simulink model "acquire_data_mag"  (R2017b)
settings: Solver=FixedStepDiscrete  StartTime=0.0  StopTime=10.0  RelTol=1e-3
undefined symbols (not defined in the file or in its folder): RGBLED_COLOR_ENUM, RGBLED_MODE_ENUM
libraries: pixhawk_slib_sensors_actuators x3
settings Model: Creator=Mr Wang  LastModifiedBy=Mr Wang
settings OptimizationCC: DefaultParameterBehavior=Inlined  MaxStackSize=128
settings DebuggingCC: ParameterTunabilityLossMsg=error
settings HardwareCC: ProdBitPerPointer=32  ProdBitPerSizeT=32  ProdBitPerPtrDiffT=32  ProdLargestAtomicInteger=Long  ProdLargestAtomicFloat=Double  ProdWordSize=32  ProdHWDeviceType=ARM Compatible->ARM Cortex
settings SFSimCC: MATLABDynamicMemAlloc=off
settings RTWCC: SystemTargetFile=ert.tlc  HardwareBoard=Pixhawk PX4  TemplateMakefile=ert_default_tmf  GenerateReport=on  Toolchain=Pixhawk Toolchain  IncludeHyperlinkInReport=on  LaunchReport=on  GenerateTraceInfo=on  GenerateTraceReport=on  GenerateTraceReportSl=on  GenerateTraceReportSf=on  GenerateTraceReportEml=on
settings CodeAppCC: ForceParamTrailComments=on  IgnoreCustomStorageClasses=off  OperatorAnnotations=on  SimulinkDataObjDesc=on  SFDataObjDesc=on  MATLABFcnDesc=on  InsertBlockDesc=on  StateflowObjectComments=on  MATLABSourceComments=on
settings ERTTargetCC: MultiwordLength=2048  ERTCustomFileTemplate=PX4_codertarget_file_process.tlc

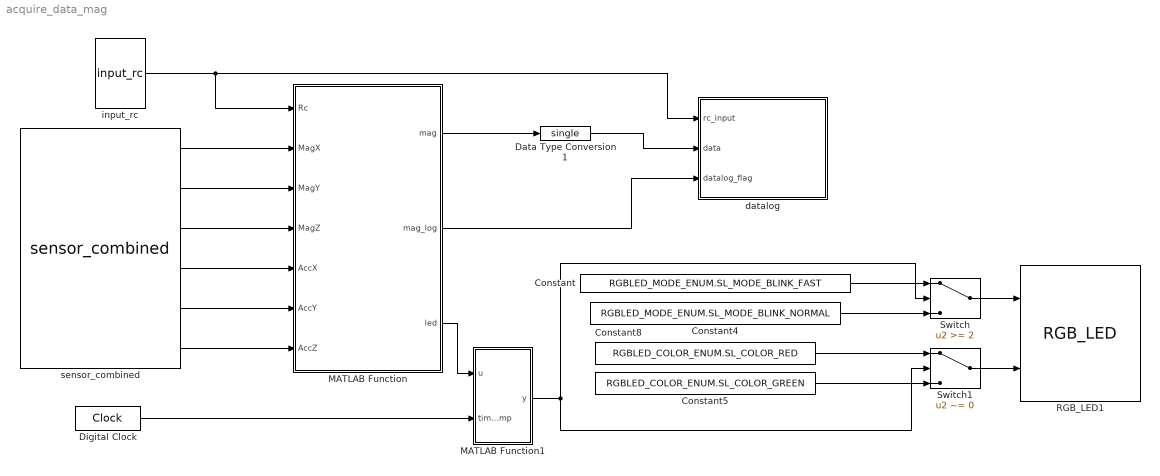
== system acquire_data_mag ==
  Constant : Constant  Value=RGBLED_MODE_ENUM.SL_MODE_BLINK_FAST  OutDataTypeStr=Enum: RGBLED_MODE_ENUM
  Constant4 : Constant  Value=RGBLED_MODE_ENUM.SL_MODE_BLINK_NORMAL  OutDataTypeStr=Enum: RGBLED_MODE_ENUM
  Constant5 : Constant  Value=RGBLED_COLOR_ENUM.SL_COLOR_GREEN  OutDataTypeStr=Enum: RGBLED_COLOR_ENUM
  Constant8 : Constant  Value=RGBLED_COLOR_ENUM.SL_COLOR_RED  OutDataTypeStr=Enum: RGBLED_COLOR_ENUM
  Data Type Conversion1 : DataTypeConversion  OutDataTypeStr=single
  Digital Clock : DigitalClock
  MATLAB Function : MATLAB Function  TreatAsAtomicUnit=on
  MATLAB Function1 : MATLAB Function  TreatAsAtomicUnit=on
  RGB_LED1 : pixhawk_slib_sensors_actuators/RGB_LED  Description=|
      | This block gives the user control over various lighting modes of the RGB LED available on the PX4 hardware. 
      | This block accepts 2 inputs: Mode and Color.  These are enumeration data types.  You can find out what values are valid in the MATLAB command window by typing: 
      | Enumeration members for class 'RGBLED_COLOR_ENUM':
      |     SL_COLOR_OFF
      |     SL_COLOR_RED
      |     SL_COLOR_GREEN
      |     SL_COLOR_BLUE
      |     SL_COLOR_YELLOW
      |     SL_COLOR_PURPLE
      |     SL_COLOR_AMBER
      |     SL_COLOR_CYAN
      |     SL_COLOR_WHITE 
      | Enumeration members for class 'RGBLED_MODE_ENUM':
      |     SL_MODE_OFF
      |     SL_MODE_ON
      |     SL_MODE_DISABLED
      |     SL_MODE_BLINK_SLOW
      |     SL_MODE_BLINK_NORMAL
      |     SL_MODE_BLINK_FAST
      |     SL_MODE_BREATHE  
      | Look at the sample Simulink model: px4demo_rgbled.slx for an example of how to use this block.
      settings: SourceProductName=Pixhawk Target Blocks
  Switch : Switch  Threshold=2
  Switch1 : Switch  Criteria=u2 ~= 0  Threshold=1500
  datalog : Subsystem
  input_rc : pixhawk_slib_sensors_actuators/input_rc  sampletime=1/250  channel1=off  channel2=off  channel3=off  channel4=off  channel5=on  channel6=off  channel7=off  channel8=off  channel9=off  channel10=off  channel11=off  channel12=off  channel13=off  channel14=off  channel15=off  channel16=off  channel17=off  channel18=off  ch_count=off  rssi=off  rc_failsafe=off  rc_lost=off  rc_inputsource=off
      settings: SourceProductName=Pixhawk Target Blocks
  sensor_combined : pixhawk_slib_sensors_actuators/sensor_combined  Description=|  sampletime=1/250  show_mag=on  show_acc=on  show_gyro=off  show_baro=off  show_ts=off
      | Sensor Combined Block
      | 
      | This block enables access to the various sensors available on the px4fmu-v2 hardware.  
      | The user can use these signals in the Simulink control model.  
      | The sample time needs to be provided in the mask dialog.  
      | Optional output ports can also be selected.  
      | Refer to the sample model: px4demo_attitude_control.slx
      | 
      | Signal definitions: 
      | Magnetometer (x,y,z) - single values – Magnetic field in NED body frame, in Gauss 
      | Accelerometer (x,y,z) - single values – Acceleration in NED body frame, in m/s^2 
      | Gyroscope (p,q,r) - single values – Angular velocity in radians per second 
      | Barometer (Altitude) - single value – Barometric pressure, already temperature compensated (millibars) 
      | RunTime (timestamp) - double value – Timestamp in microseconds since boot, from gyro 
      |   
      | The sensor_combined block needs to have the px4io service running on the PX4 hardware in order to get valid signal values.
      settings: SourceProductName=Pixhawk Target Blocks
  wires:
  input_rc/1 -> MATLAB Function/1(Rc), datalog/1(rc_input)
  sensor_combined/1 -> MATLAB Function/2(MagX)
  sensor_combined/2 -> MATLAB Function/3(MagY)
  sensor_combined/3 -> MATLAB Function/4(MagZ)
  MATLAB Function/1(mag) -> Data Type Conversion1/1
  Data Type Conversion1/1 -> datalog/2(data)
  MATLAB Function/2(mag_log) -> datalog/3(datalog_flag)
  sensor_combined/4 -> MATLAB Function/5(AccX)
  sensor_combined/5 -> MATLAB Function/6(AccY)
  sensor_combined/6 -> MATLAB Function/7(AccZ)
  MATLAB Function/3(led) -> MATLAB Function1/1(u)
  Digital Clock/1 -> MATLAB Function1/2(timestamp)
  Constant8/1 -> Switch1/1
  Constant5/1 -> Switch1/3
  Switch/1 -> RGB_LED1/1
  Constant4/1 -> Switch/3
  MATLAB Function1/1(y) -> Switch/2, Switch1/2
  Switch1/1 -> RGB_LED1/2
  Constant/1 -> Switch/1

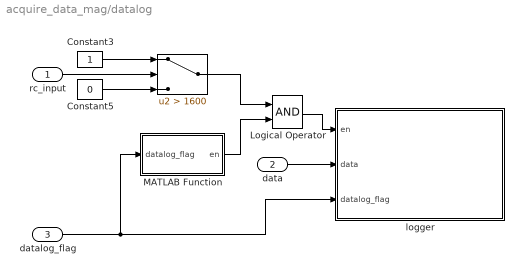
== system acquire_data_mag/datalog ==
  rc_input : Inport
  data : Inport  Port=2
  datalog_flag : Inport  Port=3
  " " : Switch  Criteria=u2 > Threshold  Threshold=1600
  Constant3 : Constant
  Constant5 : Constant  Value=0
  Logical Operator : Logic  AllPortsSameDT=off  OutDataTypeStr=boolean
  MATLAB Function : MATLAB Function  TreatAsAtomicUnit=on
  logger : Subsystem  mask(Binary Logger){logfile=/fs/microsd/log/e3_m, cacheflag=off, numRecs=1000}
      mask prompts: cacheflag "Cache in Memory"; numRecs "Max Record Count"
      mask help:
      | Log a vector of data to a file on the SD card
      |
      | If Cache in Memory is on data is written when en goes low or when max number of records specified is reached.
      | Otherwise Max Number of Records is used to indicate when to performa an fflush out to file.
      mask init:
      | logname=uint8(logfile);
      mask Help: eval('pixhawk.internal.doc(''binary_logger_Block.html'')');
      mask Display:
      | fprintf(get_param(gcb,'logfile'))
      | port_label('input',1,'en')
      | port_label('input',2,'data')
      | port_label('input',3,'datalog_flag')
  wires:
  rc_input/1 -> " "/2
  data/1 -> logger/2(data)
  datalog_flag/1 -> logger/3(datalog_flag), MATLAB Function/1(datalog_flag)
  Constant3/1 -> " "/1
  Constant5/1 -> " "/3
  " "/1 -> Logical Operator/1
  MATLAB Function/1(en) -> Logical Operator/2
  Logical Operator/1 -> logger/1(en)

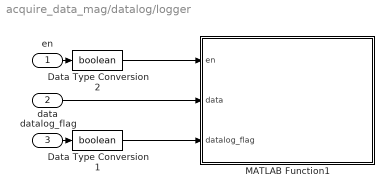
== system acquire_data_mag/datalog/logger ==
  en : Inport
  data : Inport  Port=2
  datalog_flag : Inport  Port=3
  Data Type Conversion1 : DataTypeConversion  OutDataTypeStr=boolean
  Data Type Conversion2 : DataTypeConversion  OutDataTypeStr=boolean
  MATLAB Function1 : MATLAB Function  TreatAsAtomicUnit=on
  wires:
  data/1 -> MATLAB Function1/2(data)
  Data Type Conversion2/1 -> MATLAB Function1/1(en)
  en/1 -> Data Type Conversion2/1
  datalog_flag/1 -> Data Type Conversion1/1
  Data Type Conversion1/1 -> MATLAB Function1/3(datalog_flag)

== matlab function acquire_data_mag/datalog/logger/MATLAB Function1 ==
  data: en input boolean; data input; datalog_flag input boolean; logname parameter uint8; cacheflag parameter boolean; numRecs parameter uint32
%% Binary Logger
% Note: All data needs to be of the same type (e.g. double)
% Header information format:
%           String "MWLOGV##"
%           Time/Date 4 bytes (time())
%           Number of Signals per record Logged 1 byte (256 max)
%           Data Type of Signals Logged  1 byte (1-10)
%           Number of bytes per record 2 bytes (65535 max)
% This does NOT include the number of data sets logged.  
% i.e. The Reader is responsible for reading until EOF.
% MathWorks Pilot Engineering 2015
% Steve Kuznicki
function binary_logger(en, data, datalog_flag, logname, cacheflag, numRecs)
%#codegen
    persistent fp isflushed isopen count lognumstr elem_size vect_size
    coder.cinclude('<stdio.h>');
    coder.cinclude('<time.h>');
    
    if isempty(count)
        count = uint32(0);
        lognumstr = 65;
        isopen = false;
        fp = coder.opaque('FILE*', 'NULL');
        isflushed = false;
        elem_size = uint16(1);
        vect_size = coder.const(uint8(numel(data)));
        if cacheflag == true
            %datastored = zeros(numRecs*uint32(coder.const(numel(data))), 1, 'like', data);
        end
    end

    if (en)
        if isopen == false
            [elsize, eltype] = get_elem_size(data);
            elem_size = coder.const(uint16(elsize));
            elem_type = coder.const(uint8(eltype));
            vect_size = coder.const(uint8(numel(data)));
            coder.ceval('printf',['OPENING file %s vect_size %d elem_size %d numRecs %d %c' uint8(0)], ...
                [logname, '_', char(lognumstr), '.bin', int8(0)], uint32(vect_size), uint32(elem_size), uint32(numRecs), uint8(10));
            fp = coder.ceval('fopen', [logname, '_', char(lognumstr), '.bin', int8(0)], ['wb', int8(0)]);
            lognumstr = lognumstr + 1;
            isflushed = false;
            count = uint32(0);
            isopen = true;
            % Write header information here
            % header token + version
            mlStrVer = 'MWLOGV01';
            coder.ceval('fwrite', coder.rref(mlStrVer), uint32(1), length(mlStrVer), fp);
            % date/time
            tm = uint32(0);
            tmptr = uint32(0);
            tm = coder.ceval('time',coder.wref(tmptr));
            coder.ceval('fwrite', coder.rref(tm), uint32(4), uint32(1), fp);
            % number of elements in each record
            coder.ceval('fwrite', coder.rref(vect_size), uint32(1), uint32(1), fp);
            % data type of the elements
            coder.ceval('fwrite', coder.rref(elem_type), uint32(1), uint32(1), fp);
            % size of each record in bytes
            recSize = elem_size * uint16(vect_size);
            coder.ceval('fwrite', coder.rref(recSize), uint32(2), uint32(1), fp);
        end
        % cache data in memory or use fwrite
        if cacheflag == true
            addr = (count*uint32(vect_size))+1;
            for idx = 1:vect_size
                %datastored(addr) = data(idx);
                addr = addr + 1;
            end
            count = count + uint32(1);
        else
            if  datalog_flag
                coder.ceval('fwrite', coder.rref(data), elem_size, vect_size, fp);
                count = count + uint32(1);
            end
        end
        
        % check for data count limit
        if count >= numRecs
            if cacheflag
                for idx = 1:count*uint32(vect_size)
                    %coder.ceval('fwrite', coder.rref(datastored(idx)), elem_size, uint32(1), fp);
                end
            end
            coder.ceval('fflush', fp);
            isflushed = false;
            count = uint32(0);
        end
    else
        if isopen == true
            if ~isflushed 
                coder.ceval('printf',['CLOSING file. count = %d %c' uint8(0)], uint32(count), uint8(10));
                if cacheflag
                    count = count + uint32(1);
                    for idx = 1:count*uint32(vect_size)
                        %coder.ceval('fwrite', coder.rref(datastored(idx)), elem_size, uint32(1), fp);
                    end
                end
                coder.ceval('fflush', fp);
                isflushed = true;
            end
            coder.ceval('fclose', fp);
        end
        isopen = false;
        count = uint32(0);
    end
end

% return the size of the element in bytes
function [elem_size, dtype] = get_elem_size(data)
    switch(class(data))
        case 'double'
            elem_size = 8;
            dtype = 1;
        case 'single'
            elem_size = 4;
            dtype = 2;
        case 'int32'
            elem_size = 4;
            dtype = 3;
        case 'uint32'
            elem_size = 4;
            dtype = 4;
        case 'int16'
            elem_size = 2;
            dtype = 5;
        case 'uint16'
            elem_size = 2;
            dtype = 6;
        case 'int8'
            elem_size = 1;
            dtype = 7;
        case 'uint8'
            elem_size = 1;
            dtype = 8;
        case 'logical'
            elem_size = 1;
            dtype = 9;
        case 'embedded.fi'
            nt = numerictype(data);
            elem_size = 2^ceil(log2(ceil(nt.WordLength / 8)));
            dtype = 10;
    end
    if ~isreal(data)
        elem_size = elem_size*2;
    end
    
    elem_size = uint16(elem_size);
    dtype = uint8(dtype);
end

== matlab function acquire_data_mag/MATLAB Function ==
  data: Rc input; MagX input; MagY input; MagZ input; AccX input; AccY input; AccZ input; mag output; mag_log output; led output
function [mag, mag_log, led]  = fcn(Rc, MagX ,MagY, MagZ, AccX ,AccY, AccZ)
%Function description:
%  Collect data for magnetometer calibration. The collected data includes
%  the feature points. The principle of selecting feature points is that  the
%  distance from all previous feature points is greater than _mindist_.
%Input:
%  rc: the remote control input, in the range of 1000-2000, and when rc >
%       1600, start collecting data. 
%  MagX ,MagY, MagZ, AccX ,AccY, AccZ: the value of the magnetometer and accelerometer read
%                                from the IMU, in Gs, m/s2 respectively. 
%Output:
%  mag: 3-dimensional array, feature points.
%  mag_log：If a feature point is collected mag_log =1,
%                               else mag_log = 0.
% led:  when one orientation is done led = 1; all six orientation is done
%        led = 2;
para_mag.oneDirectionPoints = 40; 
para_mag.maxSimplePoints = 40*6;
para_mag.mindist = 0.08*0.5;
g = 9.8;
    persistent mag_valid;
    if  isempty(mag_valid)
        mag_valid = single(zeros(3, para_mag.maxSimplePoints));
    end
    persistent mag_cal_flag
    if isempty(mag_cal_flag)
        mag_cal_flag.init = false;
        mag_cal_flag.log_finished = false;
        mag_cal_flag.faceup = false;
        mag_cal_flag.facedown = false;
        mag_cal_flag.right = false;
        mag_cal_flag.left = false;
        mag_cal_flag.noseup = false;
        mag_cal_flag.nosedown = false;
    end
   
    persistent mag_count;
    if  isempty(mag_count)
        mag_count.faceup = 0;
        mag_count.facedown = 0;
        mag_count.right = 0;
        mag_count.left = 0;
        mag_count.noseup = 0;
        mag_count.nosedown = 0;
    end
    
    persistent vcount;
    if  isempty(vcount)
        vcount = 0;
    end
    
    persistent log_finished;
    if  isempty(log_finished)
        log_finished = false;
    end
    led = 0;
    mag = single(zeros(3, 1));
    mag_log = false;
    if Rc>1600 && ~log_finished  %Manually control whether to write data
        mag = [MagX, MagY, MagZ]';
            mag_valid_flag = true;
            
            % judge direction
            if AccZ > 0.8*g && ~mag_cal_flag.faceup
                direction = 1;
            elseif AccZ < -0.8*g && ~mag_cal_flag.facedown
                 direction = 2;
            elseif AccY < -0.8*g && ~mag_cal_flag.left
                 direction = 3;
            elseif AccY > 0.8*g && ~mag_cal_flag.right
                direction = 4;
            elseif AccX > 0.8*g && ~mag_cal_flag.nosedown
                direction = 5;
            elseif AccX < -0.8*g && ~mag_cal_flag.noseup
                direction = 6;
            else
                direction = 0;
            end
            switch direction
                case 1
                    if vcount~=0
                        for k = 1:vcount % check if the distance of collected data from others is too close
                            dis = norm(mag - mag_valid(1:3, k));
                            if dis < para_mag.mindist  % discard the sample data if the distance is too close
                                 mag_valid_flag = false;
                                 break;
                            end
                        end
                        if mag_valid_flag
                            vcount = vcount+1;  % the number of feature points
                            mag_count.faceup = mag_count.faceup + 1;
                            mag_valid(1:3,vcount) = mag;
                        end
                    else
                        mag_valid_flag = true;
                        vcount = 1;  % first sample, record
                        mag_count.faceup = mag_count.faceup + 1;
                        mag_valid(1:3, vcount) = mag;
                    end
                    if mag_valid_flag
                        mag_log = true;
                    end
                    if mag_count.faceup >= para_mag.oneDirectionPoints
                        mag_cal_flag.faceup = true;
                        led = 1;
                    end
                case 2
                    if vcount~= 0
                        for k = 1:vcount 
                            dis = norm(mag - mag_valid(1:3, k));
                            if dis < para_mag.mindist 
                                 mag_valid_flag = false;
                                 break;
                            end
                        end
                        if mag_valid_flag
                            vcount = vcount+1;  
                            mag_count.facedown = mag_count.facedown + 1;
                            mag_valid(1:3, vcount) = mag; 
                        end
                    else
                        mag_valid_flag = true;
                        vcount = 1;  
                        mag_count.facedown = mag_count.facedown + 1;
                        mag_valid(1:3, vcount) = mag;
                    end
                    if mag_valid_flag
                            mag_log = true;
                    end
                    if mag_count.facedown >= para_mag.oneDirectionPoints
                        mag_cal_flag.facedown = true;
                        led = 1;
                    end
                case 3
                    if vcount ~= 0
                        for k = 1:vcount  
                            dis = norm(mag - mag_valid(1:3, k));
                            if dis < para_mag.mindist
                                 mag_valid_flag = false;
                                 break;
                            end
                        end
                        if mag_valid_flag
                            vcount = vcount+1;
                            mag_count.left = mag_count.left + 1;
                            mag_valid(1:3, vcount) = mag;
                       
                         end
                    else
                        mag_valid_flag = true;
                        vcount = 1;
                        mag_count.left = mag_count.left + 1;
                        mag_valid(1:3, vcount) = mag;
                    end
                    if mag_valid_flag
                            mag_log = true;
                    end
                   
                    if mag_count.left >= para_mag.oneDirectionPoints
                        mag_cal_flag.left = true;
                        led = 1;
                    end
                case 4
                    if vcount ~= 0
                        for k = 1:vcount
                            dis = norm(mag - mag_valid(1:3, k));
                            if dis < para_mag.mindist
                                 mag_valid_flag = false;
                                 break;
                            end
                        end
                        if mag_valid_flag
                            vcount = vcount + 1;
                            mag_count.right = mag_count.right + 1;
                            mag_valid(1:3, vcount) = mag;
                        
                         end
                    else
                        mag_valid_flag = true;
                        vcount = 1;
                        mag_count.right = mag_count.right + 1;
                        mag_valid(1:3, vcount) = mag;
                    end
                    if mag_valid_flag
                            
                            mag_log = true;
                    end
                    if mag_count.right >= para_mag.oneDirectionPoints
                        mag_cal_flag.right = true;
                        led = 1;
                    end    
                case 5
                    if vcount ~= 0
                        for k = 1:vcount
                            dis = norm(mag - mag_valid(1:3 ,k));
                            if dis < para_mag.mindist
                                 mag_valid_flag = false;
                                 break;
                            end
                        end
                        if mag_valid_flag
                            vcount = vcount + 1;
                            mag_count.nosedown = mag_count.nosedown + 1;
                            mag_valid(1:3, vcount) = mag;
                            
                        end
                    else
                        mag_valid_flag = true;
                        vcount = 1;
                        mag_count.nosedown = mag_count.nosedown + 1;
                        mag_valid(1:3, vcount) = mag;
                    end
                    if mag_valid_flag
                            mag_log = true;
                    end
                    if mag_count.nosedown >= para_mag.oneDirectionPoints
                        mag_cal_flag.nosedown = true;
                        led = 1;
                    end    
                case 6
                    if vcount ~= 0
                        for k = 1:vcount
                            dis = norm(mag - mag_valid(1:3, k));
                            if dis < para_mag.mindist
                                 mag_valid_flag = false;
                                 break;
                            end
                        end
                        if mag_valid_flag
                            vcount = vcount+1;
                            mag_count.noseup = mag_count.noseup + 1;
                            mag_valid(1:3, vcount) = mag;
                          
                        end
                    else
                        mag_valid_flag = true;
                        vcount = 1;
                        mag_count.noseup = mag_count.noseup + 1;
                        mag_valid(1:3, vcount)=mag;
                    end
                    if mag_valid_flag
                            mag_log = true;
                    end
                    if mag_count.noseup >= para_mag.oneDirectionPoints
                        mag_cal_flag.noseup = true;
                        led = 1;
                    end
                otherwise
                    led = 0;
            end
            
            if mag_cal_flag.noseup && mag_cal_flag.nosedown && mag_cal_flag.facedown && ...
                    mag_cal_flag.faceup && mag_cal_flag.left && mag_cal_flag.right
                led = 2;
                log_finished = true;
            else
                log_finished = false;
            end
    else
        led = 0;
    end
end

== matlab function acquire_data_mag/datalog/MATLAB Function ==
  data: datalog_flag input; en output
function en = fcn(datalog_flag)

persistent count;
if isempty(count)
    count=0;
end

if datalog_flag
    count=count+1;
end
if count>60000
    en = false;
    count=0;
else
    en = true;
end

== matlab function acquire_data_mag/MATLAB Function1 ==
  data: u input; y output; timestamp input
function y = fcn(u,timestamp)
persistent t;
    if  isempty(t)
        t=timestamp;
    end
    persistent led_t;
    if  isempty(led_t)
        led_t=0;
    end
    persistent a_count;
    if  isempty(a_count)
        a_count=0;
    end
    if u>0.5 
        led_t = 1;
        t=timestamp;
        a_count = a_count + 1;
    end
        
        
        if led_t > 0.5 && timestamp - t < 2
            y=1;
            if a_count >= 6
                y = 2;
            end
        else
            y=0;
            led_t = 0;
        end
end
